simulink model "zynqRadioHWSWLTEPBCHGeneratorRFSoC2x2"  (R2022a)
settings: Solver=FixedStepDiscrete  StartTime=0.0  StopTime=2*simParams.stopTime  RelTol=1e-3
PreLoadFcn:
  | zynqRadioHWSWLTEInit;
InitFcn:
  | zynqRadioHWSWLTEInit;
undefined symbols (not defined in the file): simParams, testWaveform0Data, testWaveform0Length, testWaveform1Data, testWaveform1Length, testWaveform2Data, testWaveform2Length
libraries: dsphdlfiltering2 x8, dspmlti4 x3, hdlsllib x3, xilinxrfsoclib x2
settings Model: DataTypeOverride=Off  SimulationMode=accelerator  Creator=The MathWorks, Inc.  LastModifiedBy=pshubh
settings SolverCC: AlgebraicLoopSolver=TrustRegion
settings DataIOCC: LimitDataPoints=on  SaveFormat=Array  SaveOutput=off  VisualizeSimOutput=off  SaveTime=off  ReturnWorkspaceOutputs=off
settings OptimizationCC: BlockReduction=off  BooleanDataType=off  ConditionallyExecuteInputs=off  DefaultParameterBehavior=Inlined  InheritOutputTypeSmallerThanSingle=on  EfficientMapNaN2IntZero=off  LifeSpan=inf
settings DebuggingCC: AlgebraicLoopMsg=error  SaveWithParameterizedLinksMsg=none  UnderspecifiedInitializationDetection=Classic  MergeDetectMultiDrivingBlocksExec=none  SignalResolutionControl=TryResolveAllWithWarning  InheritedTsInSrcMsg=none  SingleTaskRateTransMsg=error  ParameterPrecisionLossMsg=none  UnconnectedInputMsg=warning  UnconnectedOutputMsg=warning  UnconnectedLineMsg=warning  AllowSymbolicDim=off  StrictBusMsg=ErrorOnBusTreatedAsVector  SFUnexpectedBacktrackingDiag=warning  SFNoUnconditionalDefaultTransitionDiag=warning  SFExecutionAtInitializationDiag=none  SFMachineParentedDataDiag=warning  ArithmeticOperatorsInVariantConditions=warning
settings HardwareCC: ProdBitPerPointer=32  ProdBitPerSizeT=32  ProdBitPerPtrDiffT=32  ProdLargestAtomicFloat=None  ProdIntDivRoundTo=Undefined  ProdEndianess=Unspecified  ProdWordSize=32  ProdHWDeviceType=ASIC/FPGA->ASIC/FPGA  TargetBitPerPointer=64  TargetBitPerSizeT=64  TargetBitPerPtrDiffT=64  TargetLongLongMode=on  TargetIntDivRoundTo=Zero  TargetEndianess=LittleEndian  TargetWordSize=64  TargetHWDeviceType=MATLAB Host  ProdEqTarget=off
settings ModelReferenceCC: UpdateModelReferenceTargets=IfOutOfDate  PropagateSignalLabelsOutOfModel=off
settings SFSimCC: SimUseLocalCustomCode=off
settings RTWCC: RTWUseLocalCustomCode=off
settings CodeAppCC: MaxIdLength=128  StateflowObjectComments=on
settings GRTTargetCC: TargetLangStandard=C89/C90 (ANSI)  CombineOutputUpdateFcns=off  GRTInterface=on
settings ConfigComp: CovMetricSettings=dw  CovSaveCumulativeToWorkspaceVar=on  CovSaveSingleToWorkspaceVar=on  CovExternalEMLEnable=off  CovSFcnEnable=off

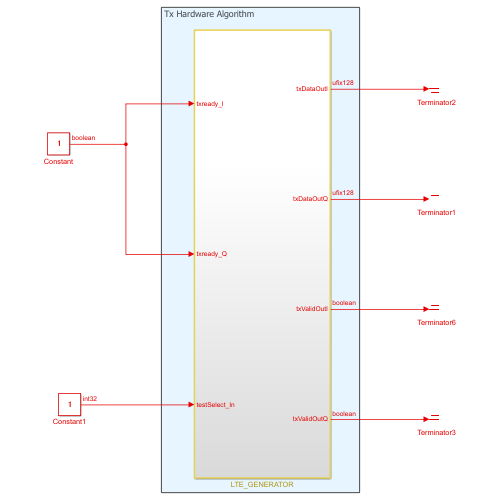
[thumbnail: Simulink's stored preview of the top-level diagram]
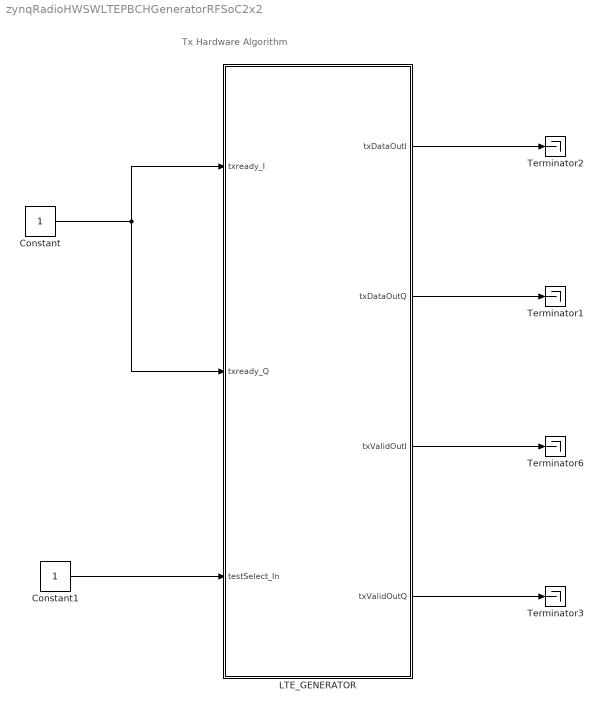
== system zynqRadioHWSWLTEPBCHGeneratorRFSoC2x2 ==
  note: Tx Hardware Algorithm
  Constant : Constant  VectorParams1D=off  OutDataTypeStr=boolean  SampleTime=simParams.Ts
  Constant1 : Constant  VectorParams1D=off  OutDataTypeStr=int32  SampleTime=simParams.Ts
  LTE_GENERATOR : Subsystem  TreatAsAtomicUnit=on
  Terminator{1..3,6} (4 alike) : Terminator
  wires:
  LTE_GENERATOR/2(txDataOutQ) -> Terminator1/1
  LTE_GENERATOR/1(txDataOutI) -> Terminator2/1
  LTE_GENERATOR/4(txValidOutQ) -> Terminator3/1
  LTE_GENERATOR/3(txValidOutI) -> Terminator6/1
  Constant/1 -> LTE_GENERATOR/2(txready_Q), LTE_GENERATOR/1(txready_I)
  Constant1/1 -> LTE_GENERATOR/3(testSelect_In)

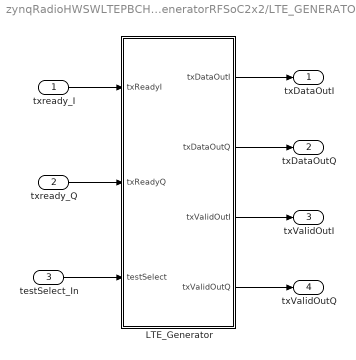
== system zynqRadioHWSWLTEPBCHGeneratorRFSoC2x2/LTE_GENERATOR ==
  txready_I : Inport
  txready_Q : Inport  Port=2
  testSelect_In : Inport  Port=3
  LTE_Generator : Subsystem
  txDataOutI : Outport  VectorParamsAs1DForOutWhenUnconnected=off
  txDataOutQ : Outport  Port=2  VectorParamsAs1DForOutWhenUnconnected=off
  txValidOutI : Outport  Port=3  VectorParamsAs1DForOutWhenUnconnected=off
  txValidOutQ : Outport  Port=4  VectorParamsAs1DForOutWhenUnconnected=off
  wires:
  LTE_Generator/2(txDataOutQ) -> txDataOutQ/1
  LTE_Generator/1(txDataOutI) -> txDataOutI/1
  LTE_Generator/4(txValidOutQ) -> txValidOutQ/1
  LTE_Generator/3(txValidOutI) -> txValidOutI/1
  txready_I/1 -> LTE_Generator/1(txReadyI)
  txready_Q/1 -> LTE_Generator/2(txReadyQ)
  testSelect_In/1 -> LTE_Generator/3(testSelect)

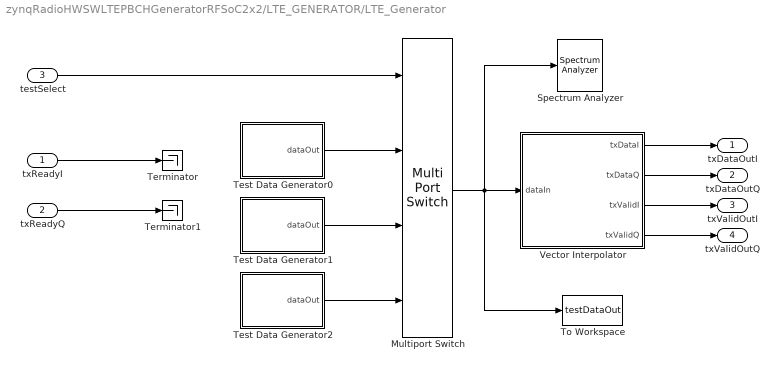
== system zynqRadioHWSWLTEPBCHGeneratorRFSoC2x2/LTE_GENERATOR/LTE_Generator ==
  txReadyI : Inport
  txReadyQ : Inport  Port=2
  testSelect : Inport  Port=3
  Multiport Switch : MultiPortSwitch  DataPortOrder=Zero-based contiguous  DiagnosticForDefault=None  zeroidx=on  SaturateOnIntegerOverflow=off  InputSameDT=off
  Spectrum Analyzer : SpectrumAnalyzer
  Terminator : Terminator
  Terminator1 : Terminator
  Test Data Generator0 : Subsystem  mask{framesBetweenStarts=400}
      mask prompts: framesBetweenStarts "Number of frames between start pulses"
      mask DialogControl Control2 Prompt: (min number of frames is 2)
  Test Data Generator1 : Subsystem  mask{framesBetweenStarts=400}
      mask prompts: framesBetweenStarts "Number of frames between start pulses"
      mask DialogControl Control2 Prompt: (min number of frames is 2)
  Test Data Generator2 : Subsystem  mask{framesBetweenStarts=400}
      mask prompts: framesBetweenStarts "Number of frames between start pulses"
      mask DialogControl Control2 Prompt: (min number of frames is 2)
  To Workspace : ToWorkspace  VariableName=testDataOut  SaveFormat=Structure With Time  SampleTime=-1
      settings: Save2DSignal=2-D array (concatenate along first dimension)
  Vector Interpolator : Subsystem  TreatAsAtomicUnit=on
  txDataOutI : Outport  VectorParamsAs1DForOutWhenUnconnected=off
  txDataOutQ : Outport  Port=2  VectorParamsAs1DForOutWhenUnconnected=off
  txValidOutI : Outport  Port=3  VectorParamsAs1DForOutWhenUnconnected=off
  txValidOutQ : Outport  Port=4  VectorParamsAs1DForOutWhenUnconnected=off
  wires:
  Vector Interpolator/2(txDataQ) -> txDataOutQ/1
  Vector Interpolator/1(txDataI) -> txDataOutI/1
  Vector Interpolator/3(txValidI) -> txValidOutI/1
  Vector Interpolator/4(txValidQ) -> txValidOutQ/1
  txReadyI/1 -> Terminator/1
  txReadyQ/1 -> Terminator1/1
  Multiport Switch/1 -> To Workspace/1, Spectrum Analyzer/1, Vector Interpolator/1(dataIn)
  Test Data Generator0/1(dataOut) -> Multiport Switch/2
  Test Data Generator1/1(dataOut) -> Multiport Switch/3
  Test Data Generator2/1(dataOut) -> Multiport Switch/4
  testSelect/1 -> Multiport Switch/1

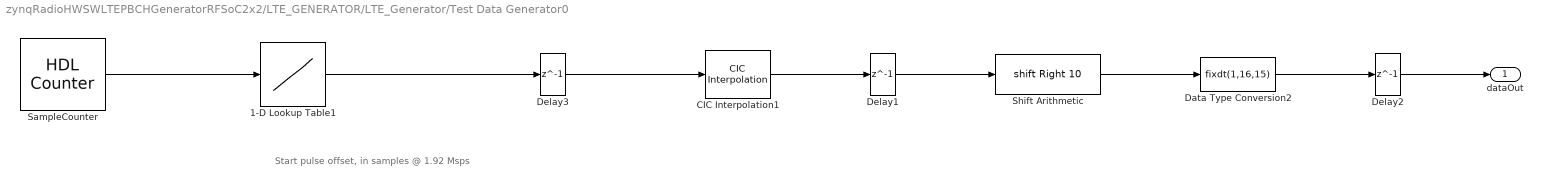
== system zynqRadioHWSWLTEPBCHGeneratorRFSoC2x2/LTE_GENERATOR/LTE_Generator/Test Data Generator0 ==
  note: Start pulse offset, in samples @ 1.92 Msps
  1-D Lookup Table1 : Lookup_n-D  NumberOfTableDimensions=1  BreakpointsSpecification=Even spacing  BreakpointsForDimension1=[-5:5]  BreakpointsForDimension1FirstPoint=0  BreakpointsForDimension2FirstPoint=10  BreakpointsForDimension2Spacing=12  IndexSearchMethod=Evenly spaced points  Table=testWaveform0Data  TableDataTypeStr=testWaveform0Data.numerictype  InterpMethod=Flat  DiagnosticForOutOfRangeInput=Error  InternalRulePriority=Speed  OutDataTypeStr=testWaveform0Data.numerictype  RndMeth=Simplest
  CIC Interpolation1 : dspmlti4/CIC Interpolation  filtFrom=Dialog parameters  filtobj=Hm_interp  ftype=Interpolator  R=32  M=1  N=3  filterInternals=Full precision  BPS=[16 16 16 16]  FLPS=0  outputWordLength=32  outputFracLength=0  launchFVT=off  framing=Allow multirate processing  OutputFrames=off
      settings: SourceProductBaseCode=DS
  Data Type Conversion2 : DataTypeConversion  OutDataTypeStr=fixdt(1,16,15)  SaturateOnIntegerOverflow=off  RndMeth=Floor
  Delay1 : Delay  DelayLength=1  InitialCondition=0  UseCircularBuffer=on
  Delay2 : Delay  DelayLength=1  InitialCondition=0  UseCircularBuffer=on
  Delay3 : Delay  DelayLength=1  InitialCondition=0  UseCircularBuffer=on
  SampleCounter : hdlsllib/Sources/HDL Counter  CountType=Count limited  CountInit=0  CountStep=1  CountMax=testWaveform0Length-1  CountFromType=Initial value  CountFrom=0  CountResetPort=off  CountLoadPort=off  CountEnbPort=off  CountDirPort=off  CountHitOutputPort=off  CountDataType=Unsigned  CountWordLen=nextpow2(testWaveform0Length)  CountFracLen=0  CountSampTime=32 * simParams.Ts
  Shift Arithmetic : ArithShift  BitShiftNumber=10  BitShiftDirection=Right
  dataOut : Outport  VectorParamsAs1DForOutWhenUnconnected=off
  wires:
  Data Type Conversion2/1 -> Delay2/1
  CIC Interpolation1/1 -> Delay1/1
  Shift Arithmetic/1 -> Data Type Conversion2/1
  SampleCounter/1 -> 1-D Lookup Table1/1
  1-D Lookup Table1/1 -> Delay3/1
  Delay3/1 -> CIC Interpolation1/1
  Delay1/1 -> Shift Arithmetic/1
  Delay2/1 -> dataOut/1

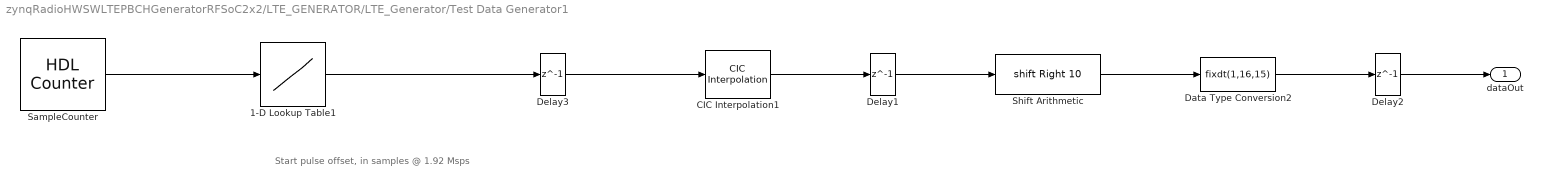
== system zynqRadioHWSWLTEPBCHGeneratorRFSoC2x2/LTE_GENERATOR/LTE_Generator/Test Data Generator1 ==
  note: Start pulse offset, in samples @ 1.92 Msps
  1-D Lookup Table1 : Lookup_n-D  NumberOfTableDimensions=1  BreakpointsSpecification=Even spacing  BreakpointsForDimension1=[-5:5]  BreakpointsForDimension1FirstPoint=0  BreakpointsForDimension2FirstPoint=10  BreakpointsForDimension2Spacing=12  IndexSearchMethod=Evenly spaced points  Table=testWaveform1Data  TableDataTypeStr=testWaveform1Data.numerictype  InterpMethod=Flat  DiagnosticForOutOfRangeInput=Error  InternalRulePriority=Speed  OutDataTypeStr=testWaveform1Data.numerictype  RndMeth=Simplest
  CIC Interpolation1 : dspmlti4/CIC Interpolation  filtFrom=Dialog parameters  filtobj=Hm_interp  ftype=Interpolator  R=32  M=1  N=3  filterInternals=Full precision  BPS=[16 16 16 16]  FLPS=0  outputWordLength=32  outputFracLength=0  launchFVT=off  framing=Allow multirate processing  OutputFrames=off
      settings: SourceProductBaseCode=DS
  Data Type Conversion2 : DataTypeConversion  OutDataTypeStr=fixdt(1,16,15)  SaturateOnIntegerOverflow=off  RndMeth=Floor
  Delay1 : Delay  DelayLength=1  InitialCondition=0  UseCircularBuffer=on
  Delay2 : Delay  DelayLength=1  InitialCondition=0  UseCircularBuffer=on
  Delay3 : Delay  DelayLength=1  InitialCondition=0  UseCircularBuffer=on
  SampleCounter : hdlsllib/Sources/HDL Counter  CountType=Count limited  CountInit=0  CountStep=1  CountMax=testWaveform1Length-1  CountFromType=Initial value  CountFrom=0  CountResetPort=off  CountLoadPort=off  CountEnbPort=off  CountDirPort=off  CountHitOutputPort=off  CountDataType=Unsigned  CountWordLen=nextpow2(testWaveform1Length)  CountFracLen=0  CountSampTime=32 * simParams.Ts
  Shift Arithmetic : ArithShift  BitShiftNumber=10  BitShiftDirection=Right
  dataOut : Outport  VectorParamsAs1DForOutWhenUnconnected=off
  wires:
  Data Type Conversion2/1 -> Delay2/1
  CIC Interpolation1/1 -> Delay1/1
  Shift Arithmetic/1 -> Data Type Conversion2/1
  SampleCounter/1 -> 1-D Lookup Table1/1
  1-D Lookup Table1/1 -> Delay3/1
  Delay3/1 -> CIC Interpolation1/1
  Delay1/1 -> Shift Arithmetic/1
  Delay2/1 -> dataOut/1

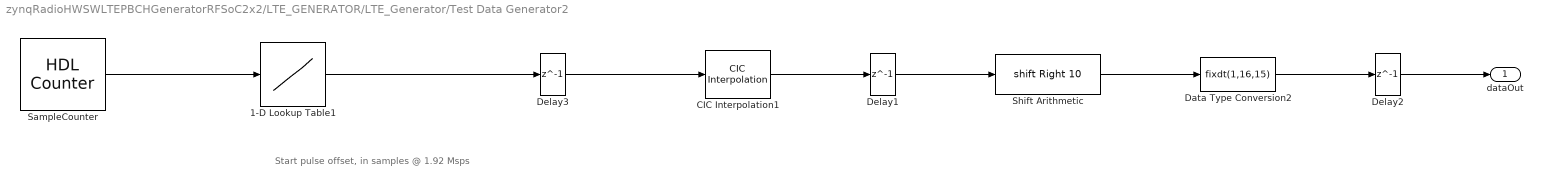
== system zynqRadioHWSWLTEPBCHGeneratorRFSoC2x2/LTE_GENERATOR/LTE_Generator/Test Data Generator2 ==
  note: Start pulse offset, in samples @ 1.92 Msps
  1-D Lookup Table1 : Lookup_n-D  NumberOfTableDimensions=1  BreakpointsSpecification=Even spacing  BreakpointsForDimension1=[-5:5]  BreakpointsForDimension1FirstPoint=0  BreakpointsForDimension2FirstPoint=10  BreakpointsForDimension2Spacing=12  IndexSearchMethod=Evenly spaced points  Table=testWaveform2Data  TableDataTypeStr=testWaveform2Data.numerictype  InterpMethod=Flat  DiagnosticForOutOfRangeInput=Error  InternalRulePriority=Speed  OutDataTypeStr=testWaveform2Data.numerictype  RndMeth=Simplest
  CIC Interpolation1 : dspmlti4/CIC Interpolation  filtFrom=Dialog parameters  filtobj=Hm_interp  ftype=Interpolator  R=32  M=1  N=3  filterInternals=Full precision  BPS=[16 16 16 16]  FLPS=0  outputWordLength=32  outputFracLength=0  launchFVT=off  framing=Allow multirate processing  OutputFrames=off
      settings: SourceProductBaseCode=DS
  Data Type Conversion2 : DataTypeConversion  OutDataTypeStr=fixdt(1,16,15)  SaturateOnIntegerOverflow=off  RndMeth=Floor
  Delay1 : Delay  DelayLength=1  InitialCondition=0  UseCircularBuffer=on
  Delay2 : Delay  DelayLength=1  InitialCondition=0  UseCircularBuffer=on
  Delay3 : Delay  DelayLength=1  InitialCondition=0  UseCircularBuffer=on
  SampleCounter : hdlsllib/Sources/HDL Counter  CountType=Count limited  CountInit=0  CountStep=1  CountMax=testWaveform2Length-1  CountFromType=Initial value  CountFrom=0  CountResetPort=off  CountLoadPort=off  CountEnbPort=off  CountDirPort=off  CountHitOutputPort=off  CountDataType=Unsigned  CountWordLen=nextpow2(testWaveform2Length)  CountFracLen=0  CountSampTime=32 * simParams.Ts
  Shift Arithmetic : ArithShift  BitShiftNumber=10  BitShiftDirection=Right
  dataOut : Outport  VectorParamsAs1DForOutWhenUnconnected=off
  wires:
  Data Type Conversion2/1 -> Delay2/1
  CIC Interpolation1/1 -> Delay1/1
  Shift Arithmetic/1 -> Data Type Conversion2/1
  SampleCounter/1 -> 1-D Lookup Table1/1
  1-D Lookup Table1/1 -> Delay3/1
  Delay3/1 -> CIC Interpolation1/1
  Delay1/1 -> Shift Arithmetic/1
  Delay2/1 -> dataOut/1

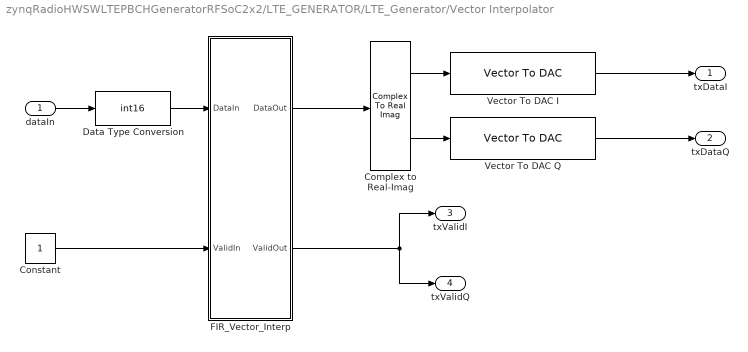
== system zynqRadioHWSWLTEPBCHGeneratorRFSoC2x2/LTE_GENERATOR/LTE_Generator/Vector Interpolator ==
  dataIn : Inport
  Complex to Real-Imag : ComplexToRealImag
  Constant : Constant  OutDataTypeStr=boolean  SampleTime=simParams.Ts
  Data Type Conversion : DataTypeConversion  OutDataTypeStr=int16  ConvertRealWorld=Stored Integer (SI)  SaturateOnIntegerOverflow=off  RndMeth=Floor
  FIR_Vector_Interp : Subsystem
  Vector To DAC I : xilinxrfsoclib/Vector To DAC  INPUT_WL=16  DT_INPUT=0
      settings: SourceProductBaseCode=XILINX_BLOCKSET
  Vector To DAC Q : xilinxrfsoclib/Vector To DAC  INPUT_WL=16  DT_INPUT=0
      settings: SourceProductBaseCode=XILINX_BLOCKSET
  txDataI : Outport
  txDataQ : Outport  Port=2
  txValidI : Outport  Port=3
  txValidQ : Outport  Port=4
  wires:
  dataIn/1 -> Data Type Conversion/1
  FIR_Vector_Interp/2(ValidOut) -> txValidI/1, txValidQ/1
  Constant/1 -> FIR_Vector_Interp/2(ValidIn)
  FIR_Vector_Interp/1(DataOut) -> Complex to Real-Imag/1
  Complex to Real-Imag/1 -> Vector To DAC I/1
  Vector To DAC I/1 -> txDataI/1
  Vector To DAC Q/1 -> txDataQ/1
  Complex to Real-Imag/2 -> Vector To DAC Q/1
  Data Type Conversion/1 -> FIR_Vector_Interp/1(DataIn)

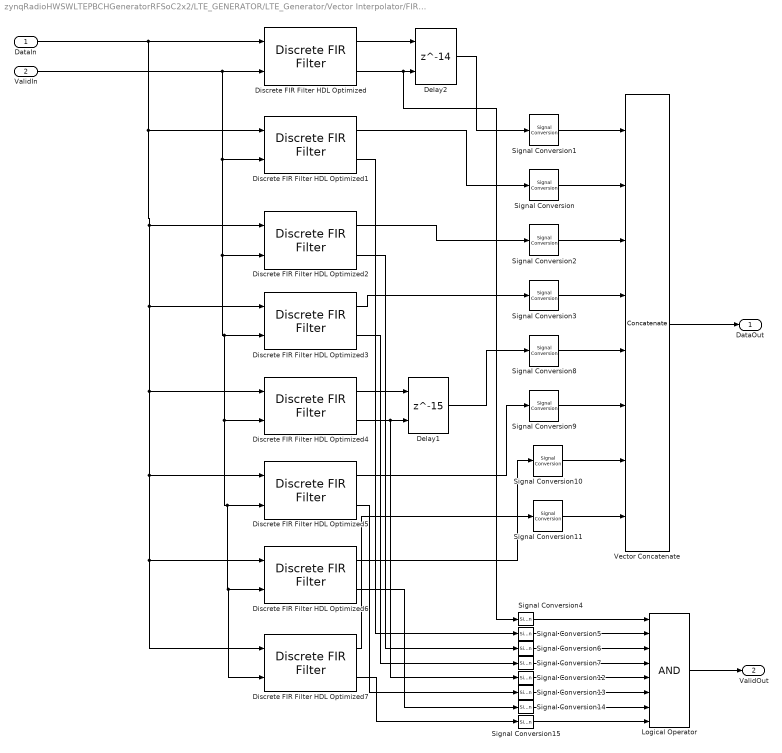
== system zynqRadioHWSWLTEPBCHGeneratorRFSoC2x2/LTE_GENERATOR/LTE_Generator/Vector Interpolator/FIR_Vector_Interp ==
  DataIn : Inport
  ValidIn : Inport  Port=2
  Delay1 : Delay  DelayLength=15  ShowEnablePort=on
      settings: InputPortMap=u0,e6
  Delay2 : Delay  DelayLength=14  ShowEnablePort=on
      settings: InputPortMap=u0,e6
  Discrete FIR Filter HDL Optimized : dsphdlfiltering2/Discrete FIR Filter  NumeratorSource=Property  Numerator=interp_coeff(1:8:end)  NumeratorPrototype=[]  FilterStructure=Direct form systolic  SerializationOption=Minimum number of cycles between valid input samples  NumCycles=2  NumberOfMultipliers=2  SimulateUsing=Code generation  roundingMode=Floor  overflowMode=off  CoefficientsDataTypeStr=Inherit: Same word length as input  OutputDataTypeStr=fixdt(1,16,0)  ResetInputPort=off  HDLGlobalReset=off
      settings: SourceProductBaseCode=HS
  Discrete FIR Filter HDL Optimized1 : dsphdlfiltering2/Discrete FIR Filter  NumeratorSource=Property  Numerator=interp_coeff(2:8:end)  NumeratorPrototype=[]  FilterStructure=Direct form systolic  SerializationOption=Minimum number of cycles between valid input samples  NumCycles=2  NumberOfMultipliers=2  SimulateUsing=Code generation  roundingMode=Floor  overflowMode=off  CoefficientsDataTypeStr=Inherit: Same word length as input  OutputDataTypeStr=fixdt(1,16,0)  ResetInputPort=off  HDLGlobalReset=off
      settings: SourceProductBaseCode=HS
  Discrete FIR Filter HDL Optimized2 : dsphdlfiltering2/Discrete FIR Filter  NumeratorSource=Property  Numerator=interp_coeff(3:8:end)  NumeratorPrototype=[]  FilterStructure=Direct form systolic  SerializationOption=Minimum number of cycles between valid input samples  NumCycles=2  NumberOfMultipliers=2  SimulateUsing=Code generation  roundingMode=Floor  overflowMode=off  CoefficientsDataTypeStr=Inherit: Same word length as input  OutputDataTypeStr=fixdt(1,16,0)  ResetInputPort=off  HDLGlobalReset=off
      settings: SourceProductBaseCode=HS
  Discrete FIR Filter HDL Optimized3 : dsphdlfiltering2/Discrete FIR Filter  NumeratorSource=Property  Numerator=interp_coeff(4:8:end)  NumeratorPrototype=[]  FilterStructure=Direct form systolic  SerializationOption=Minimum number of cycles between valid input samples  NumCycles=2  NumberOfMultipliers=2  SimulateUsing=Code generation  roundingMode=Floor  overflowMode=off  CoefficientsDataTypeStr=Inherit: Same word length as input  OutputDataTypeStr=fixdt(1,16,0)  ResetInputPort=off  HDLGlobalReset=off
      settings: SourceProductBaseCode=HS
  Discrete FIR Filter HDL Optimized4 : dsphdlfiltering2/Discrete FIR Filter  NumeratorSource=Property  Numerator=interp_coeff(5:8:end)  NumeratorPrototype=[]  FilterStructure=Direct form systolic  SerializationOption=Minimum number of cycles between valid input samples  NumCycles=2  NumberOfMultipliers=2  SimulateUsing=Code generation  roundingMode=Floor  overflowMode=off  CoefficientsDataTypeStr=Inherit: Same word length as input  OutputDataTypeStr=fixdt(1,16,0)  ResetInputPort=off  HDLGlobalReset=off
      settings: SourceProductBaseCode=HS
  Discrete FIR Filter HDL Optimized5 : dsphdlfiltering2/Discrete FIR Filter  NumeratorSource=Property  Numerator=interp_coeff(6:8:end)  NumeratorPrototype=[]  FilterStructure=Direct form systolic  SerializationOption=Minimum number of cycles between valid input samples  NumCycles=2  NumberOfMultipliers=2  SimulateUsing=Code generation  roundingMode=Floor  overflowMode=off  CoefficientsDataTypeStr=Inherit: Same word length as input  OutputDataTypeStr=fixdt(1,16,0)  ResetInputPort=off  HDLGlobalReset=off
      settings: SourceProductBaseCode=HS
  Discrete FIR Filter HDL Optimized6 : dsphdlfiltering2/Discrete FIR Filter  NumeratorSource=Property  Numerator=interp_coeff(7:8:end)  NumeratorPrototype=[]  FilterStructure=Direct form systolic  SerializationOption=Minimum number of cycles between valid input samples  NumCycles=2  NumberOfMultipliers=2  SimulateUsing=Code generation  roundingMode=Floor  overflowMode=off  CoefficientsDataTypeStr=Inherit: Same word length as input  OutputDataTypeStr=fixdt(1,16,0)  ResetInputPort=off  HDLGlobalReset=off
      settings: SourceProductBaseCode=HS
  Discrete FIR Filter HDL Optimized7 : dsphdlfiltering2/Discrete FIR Filter  NumeratorSource=Property  Numerator=interp_coeff(8:8:end)  NumeratorPrototype=[]  FilterStructure=Direct form systolic  SerializationOption=Minimum number of cycles between valid input samples  NumCycles=2  NumberOfMultipliers=2  SimulateUsing=Code generation  roundingMode=Floor  overflowMode=off  CoefficientsDataTypeStr=Inherit: Same word length as input  OutputDataTypeStr=fixdt(1,16,0)  ResetInputPort=off  HDLGlobalReset=off
      settings: SourceProductBaseCode=HS
  Logical Operator : Logic  Inputs=8  IconShape=distinctive  AllPortsSameDT=off  OutDataTypeStr=boolean
  Signal Conversion{,1..15} (16 alike) : SignalConversion  OverrideOpt=off
  Vector Concatenate : Concatenate  NumInputs=8
  DataOut : Outport
  ValidOut : Outport  Port=2
  wires:
  DataIn/1 -> Discrete FIR Filter HDL Optimized7/1, Discrete FIR Filter HDL Optimized6/1, Discrete FIR Filter HDL Optimized5/1, Discrete FIR Filter HDL Optimized4/1, Discrete FIR Filter HDL Optimized3/1, Discrete FIR Filter HDL Optimized2/1, Discrete FIR Filter HDL Optimized1/1, Discrete FIR Filter HDL Optimized/1
  Delay2/1 -> Signal Conversion1/1
  Discrete FIR Filter HDL Optimized/1 -> Delay2/1
  Discrete FIR Filter HDL Optimized1/1 -> Signal Conversion/1
  Discrete FIR Filter HDL Optimized3/1 -> Signal Conversion3/1
  Discrete FIR Filter HDL Optimized2/1 -> Signal Conversion2/1
  ValidIn/1 -> Discrete FIR Filter HDL Optimized4/2, Discrete FIR Filter HDL Optimized7/2, Discrete FIR Filter HDL Optimized6/2, Discrete FIR Filter HDL Optimized5/2, Discrete FIR Filter HDL Optimized3/2, Discrete FIR Filter HDL Optimized2/2, Discrete FIR Filter HDL Optimized1/2, Discrete FIR Filter HDL Optimized/2
  Discrete FIR Filter HDL Optimized1/2 -> Signal Conversion5/1
  Discrete FIR Filter HDL Optimized/2 -> Signal Conversion4/1, Delay2/2
  Discrete FIR Filter HDL Optimized2/2 -> Signal Conversion6/1
  Discrete FIR Filter HDL Optimized3/2 -> Signal Conversion7/1
  Vector Concatenate/1 -> DataOut/1
  Signal Conversion4/1 -> Logical Operator/1
  Signal Conversion5/1 -> Logical Operator/2
  Signal Conversion6/1 -> Logical Operator/3
  Signal Conversion7/1 -> Logical Operator/4
  Logical Operator/1 -> ValidOut/1
  Discrete FIR Filter HDL Optimized4/1 -> Delay1/1
  Discrete FIR Filter HDL Optimized4/2 -> Signal Conversion12/1, Delay1/2
  Discrete FIR Filter HDL Optimized6/2 -> Signal Conversion14/1
  Delay1/1 -> Signal Conversion8/1
  Discrete FIR Filter HDL Optimized5/1 -> Signal Conversion9/1
  Discrete FIR Filter HDL Optimized6/1 -> Signal Conversion10/1
  Discrete FIR Filter HDL Optimized7/1 -> Signal Conversion11/1
  Discrete FIR Filter HDL Optimized7/2 -> Signal Conversion15/1
  Discrete FIR Filter HDL Optimized5/2 -> Signal Conversion13/1
  Signal Conversion12/1 -> Logical Operator/5
  Signal Conversion13/1 -> Logical Operator/6
  Signal Conversion14/1 -> Logical Operator/7
  Signal Conversion15/1 -> Logical Operator/8
  Signal Conversion1/1 -> Vector Concatenate/1
  Signal Conversion/1 -> Vector Concatenate/2
  Signal Conversion2/1 -> Vector Concatenate/3
  Signal Conversion3/1 -> Vector Concatenate/4
  Signal Conversion8/1 -> Vector Concatenate/5
  Signal Conversion9/1 -> Vector Concatenate/6
  Signal Conversion10/1 -> Vector Concatenate/7
  Signal Conversion11/1 -> Vector Concatenate/8
